simulink model "Lab2_Soh_Nguyen_Kho_AbdulKadir_simulink"  (R2021a)
settings: Solver=VariableStepAuto  StartTime=0.0  StopTime=40  MaxStep=0.001  RelTol=1e-3
settings Model: Creator=afayeed  LastModifiedBy=afayeed

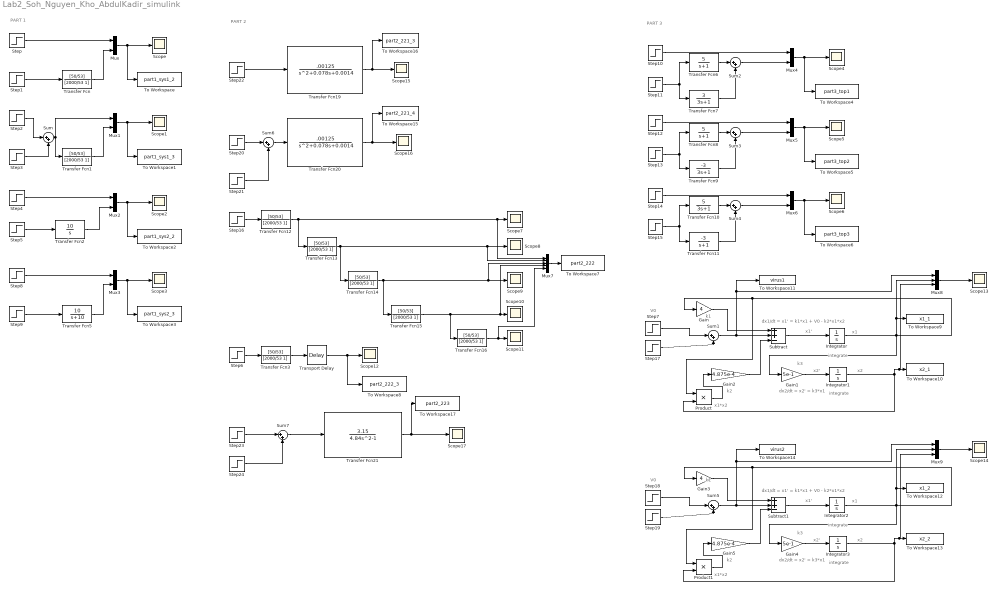
== system Lab2_Soh_Nguyen_Kho_AbdulKadir_simulink ==
  note: PART 2
  note: x1*x2
  note: dx1/dt = x1' = k1*x1 + V0 - k2*x1*x2
  note: integrate
  note: x2
  note: dx2/dt = x2' = k3*x1
  note: integrate
  note: x2'
  note: V0
  note: k2
  note: k1
  note: x1*x2
  note: x2'
  note: k3
  note: x1
  note: x1'
  note: integrate
  note: dx1/dt = x1' = k1*x1 + V0 - k2*x1*x2
  note: dx2/dt = x2' = k3*x1
  note: x2
  note: V0
  note: integrate
  note: k3
  note: x1'
  note: x1
  note: k1
  note: k2
  note: PART 1
  note: PART 3
  Gain : Gain  Gain=4
  Gain1 : Gain  Gain=5e-1
  Gain2 : Gain  Gain=4.875e-4
  Gain3 : Gain  Gain=4
  Gain4 : Gain  Gain=5e-1
  Gain5 : Gain  Gain=4.875e-4
  Integrator{,1..3} (4 alike) : Integrator
  Mux{,1..6} (7 alike) : Mux  Inputs=2
  Mux7 : Mux  Inputs=5
  Mux8 : Mux  Inputs=3
  Mux9 : Mux  Inputs=3
  Product : Product
  Product1 : Product
  Scope{,1..17} (18 alike) : Scope
  Step{,1..2,6,10..16,20,22} (13 alike) : Step  Time=0  After=10  SampleTime=0
  Step17 : Step  Time=1e-5  After=-27000  SampleTime=0
  Step18 : Step  Time=10  After=54000  SampleTime=0
  Step19 : Step  Time=10.00001  After=-54000  SampleTime=0
  Step21 : Step  Time=2  After=-10  SampleTime=0
  Step23 : Step  Time=0  After=.1  SampleTime=0
  Step24 : Step  After=-.1  SampleTime=0
  Step3 : Step  Time=2  After=-10  SampleTime=0
  Step{4..5,8..9} (4 alike) : Step  Time=0  After=0.1  SampleTime=0
  Step7 : Step  Time=0  After=27000  SampleTime=0
  Subtract : Sum  Inputs=++-
  Subtract1 : Sum  Inputs=++-
  Sum{,1..7} (8 alike) : Sum  Inputs=|++
  To Workspace : ToWorkspace  VariableName=part1_sys1_2  SampleTime=-1
  To Workspace1 : ToWorkspace  VariableName=part1_sys1_3  SampleTime=-1
  To Workspace10 : ToWorkspace  VariableName=x2_1  SampleTime=-1
  To Workspace11 : ToWorkspace  VariableName=virus1  SampleTime=-1
  To Workspace12 : ToWorkspace  VariableName=x1_2  SampleTime=-1
  To Workspace13 : ToWorkspace  VariableName=x2_2  SampleTime=-1
  To Workspace14 : ToWorkspace  VariableName=virus2  SampleTime=-1
  To Workspace15 : ToWorkspace  VariableName=part2_221_4  SampleTime=-1
  To Workspace16 : ToWorkspace  VariableName=part2_221_3  SampleTime=-1
  To Workspace17 : ToWorkspace  VariableName=part2_223  SampleTime=-1
  To Workspace2 : ToWorkspace  VariableName=part1_sys2_2  SampleTime=-1
  To Workspace3 : ToWorkspace  VariableName=part1_sys2_3  SampleTime=-1
  To Workspace4 : ToWorkspace  VariableName=part3_top1  SampleTime=-1
  To Workspace5 : ToWorkspace  VariableName=part3_top2  SampleTime=-1
  To Workspace6 : ToWorkspace  VariableName=part3_top3  SampleTime=-1
  To Workspace7 : ToWorkspace  VariableName=part2_222  SampleTime=-1
  To Workspace8 : ToWorkspace  VariableName=part2_222_3  SampleTime=-1
  To Workspace9 : ToWorkspace  VariableName=x1_1  SampleTime=-1
  Transfer Fcn{,1,3,12..16} (8 alike) : TransferFcn  Numerator=[50/53]  Denominator=[2000/53 1]
  Transfer Fcn10 : TransferFcn  Numerator=[5]  Denominator=[3 1]
  Transfer Fcn11 : TransferFcn  Numerator=[-3]  Denominator=[1 1]
  Transfer Fcn19 : TransferFcn  Numerator=[.00125]  Denominator=[1 0.078 0.0014]
  Transfer Fcn2 : TransferFcn  Numerator=[10]  Denominator=[1 0]
  Transfer Fcn20 : TransferFcn  Numerator=[.00125]  Denominator=[1 0.078 0.0014]
  Transfer Fcn21 : TransferFcn  Numerator=[3.15]  Denominator=[4.84 0 -1]
  Transfer Fcn5 : TransferFcn  Numerator=[10]  Denominator=[1 10]
  Transfer Fcn6 : TransferFcn  Numerator=[5]  Denominator=[1 1]
  Transfer Fcn7 : TransferFcn  Numerator=[3]  Denominator=[3 1]
  Transfer Fcn8 : TransferFcn  Numerator=[5]  Denominator=[1 1]
  Transfer Fcn9 : TransferFcn  Numerator=[-3]  Denominator=[3 1]
  Transport Delay : TransportDelay  DelayTime=50
  wires:
  Step1/1 -> Transfer Fcn/1
  Step/1 -> Mux/1
  Transfer Fcn/1 -> Mux/2
  Mux/1 -> To Workspace/1, Scope/1
  Step2/1 -> Sum/1
  Transfer Fcn1/1 -> Mux1/2
  Mux1/1 -> To Workspace1/1, Scope1/1
  Step3/1 -> Sum/2
  Sum/1 -> Mux1/1, Transfer Fcn1/1
  Mux2/1 -> To Workspace2/1, Scope2/1
  Step4/1 -> Mux2/1
  Step8/1 -> Mux3/1
  Transfer Fcn5/1 -> Mux3/2
  Mux3/1 -> To Workspace3/1, Scope3/1
  Step9/1 -> Transfer Fcn5/1
  Step10/1 -> Mux4/1
  Mux4/1 -> To Workspace4/1, Scope4/1
  Step11/1 -> Transfer Fcn7/1, Transfer Fcn6/1
  Transfer Fcn7/1 -> Sum2/2
  Transfer Fcn6/1 -> Sum2/1
  Mux5/1 -> To Workspace5/1, Scope5/1
  Step13/1 -> Transfer Fcn9/1, Transfer Fcn8/1
  Step12/1 -> Mux5/1
  Transfer Fcn9/1 -> Sum3/2
  Transfer Fcn8/1 -> Sum3/1
  Step15/1 -> Transfer Fcn11/1, Transfer Fcn10/1
  Transfer Fcn10/1 -> Sum4/1
  Transfer Fcn11/1 -> Sum4/2
  Mux6/1 -> To Workspace6/1, Scope6/1
  Step14/1 -> Mux6/1
  Step16/1 -> Transfer Fcn12/1
  Transfer Fcn12/1 -> Transfer Fcn13/1, Mux7/1, Scope7/1
  Transfer Fcn13/1 -> Transfer Fcn14/1, Mux7/2, Scope8/1
  Transfer Fcn14/1 -> Transfer Fcn15/1, Scope9/1, Mux7/3
  Transfer Fcn15/1 -> Transfer Fcn16/1, Mux7/4, Scope10/1
  Transfer Fcn16/1 -> Mux7/5, Scope11/1
  Step5/1 -> Transfer Fcn2/1
  Transfer Fcn2/1 -> Mux2/2
  Mux7/1 -> To Workspace7/1
  Step6/1 -> Transfer Fcn3/1
  Transfer Fcn3/1 -> Transport Delay/1
  Transport Delay/1 -> To Workspace8/1, Scope12/1
  Sum2/1 -> Mux4/2
  Sum3/1 -> Mux5/2
  Sum4/1 -> Mux6/2
  Integrator3/1 -> To Workspace13/1, Mux9/3, Product1/2
  Subtract1/1 -> Integrator2/1
  Gain1/1 -> Integrator1/1
  Step19/1 -> Sum5/2
  Sum5/1 -> Subtract1/2, To Workspace14/1, Mux9/1
  Product1/1 -> Gain5/1
  Gain2/1 -> Subtract/3
  Gain5/1 -> Subtract1/3
  Mux8/1 -> Scope13/1
  Gain4/1 -> Integrator3/1
  Integrator2/1 -> To Workspace12/1, Mux9/2, Gain4/1, Product1/1, Gain3/1
  Gain3/1 -> Subtract1/1
  Mux9/1 -> Scope14/1
  Sum1/1 -> Subtract/2, To Workspace11/1, Mux8/1
  Product/1 -> Gain2/1
  Integrator1/1 -> To Workspace10/1, Mux8/3, Product/2
  Integrator/1 -> To Workspace9/1, Mux8/2, Gain1/1, Product/1, Gain/1
  Step17/1 -> Sum1/2
  Subtract/1 -> Integrator/1
  Step18/1 -> Sum5/1
  Step7/1 -> Sum1/1
  Gain/1 -> Subtract/1
  Sum6/1 -> Transfer Fcn20/1
  Step20/1 -> Sum6/1
  Transfer Fcn20/1 -> To Workspace15/1, Scope16/1
  Transfer Fcn19/1 -> To Workspace16/1, Scope15/1
  Step21/1 -> Sum6/2
  Step22/1 -> Transfer Fcn19/1
  Step23/1 -> Sum7/1
  Sum7/1 -> Transfer Fcn21/1
  Step24/1 -> Sum7/2
  Transfer Fcn21/1 -> To Workspace17/1, Scope17/1
